simulink model "simulink_q1"  (R2022b)
settings: Solver=VariableStepAuto  StartTime=0.0  StopTime=10.0  RelTol=1e-3
settings Model: Creator=NITRO  LastModifiedBy=NITRO

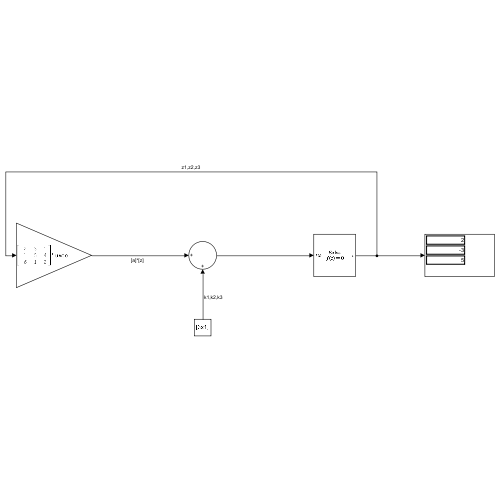
[thumbnail: Simulink's stored preview of the top-level diagram]
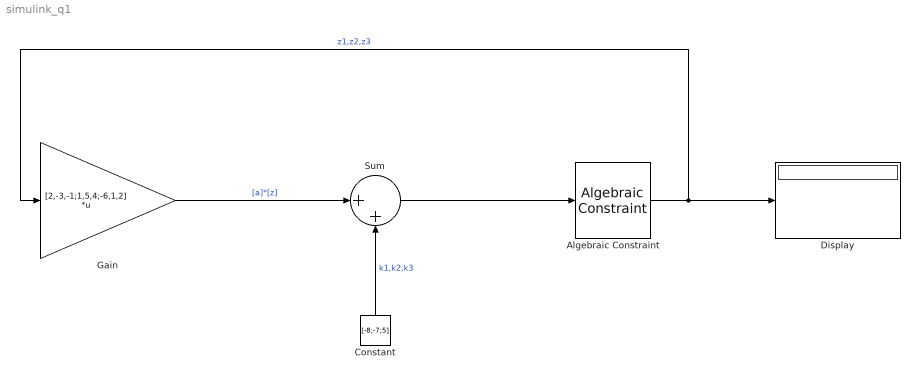
== system simulink_q1 ==
  Algebraic Constraint : AlgebraicConstraint
  Constant : Constant  Value=[-8;-7;5]
  Display : Display
  Gain : Gain  Gain=[2,-3,-1;1,5,4;-6,1,2]  Multiplication=Matrix(K*u) (u vector)
  Sum : Sum  Inputs=|++
  wires:
  Gain/1 -> Sum/1  "[a]*[z]"
  Sum/1 -> Algebraic Constraint/1
  Constant/1 -> Sum/2  "k1,k2,k3"
  Algebraic Constraint/1 -> Display/1, Gain/1  "z1,z2,z3"
